simulink model "cdm"  (R2021a)
settings: Solver=VariableStepAuto  StartTime=0.0  StopTime=10  RelTol=1e-7
values from neighbouring files (symbols this model uses):
  A = [0 1; -8.31 -6.08]    [usv.m]
  B = [0; 8.31]    [usv.m]
  C = [1 0]    [usv.m]
  K = [0 0 1]*Con    [usv.m]
settings Model: Creator=lang  LastModifiedBy=lang

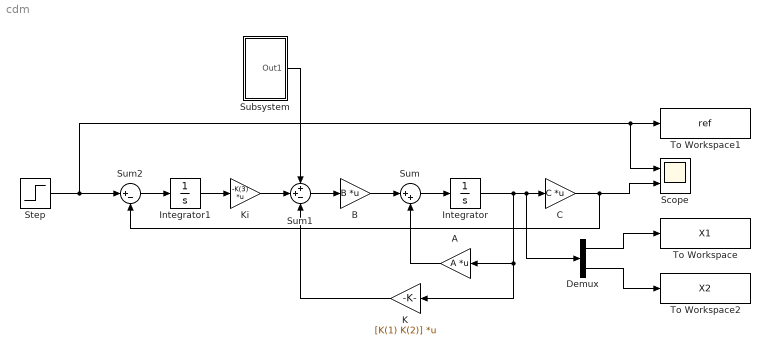
== system cdm ==
  A : Gain  Gain=A  Multiplication=Matrix(K*u)
  B : Gain  Gain=B  Multiplication=Matrix(K*u)
  C : Gain  Gain=C  Multiplication=Matrix(K*u)
  Demux : Demux  Outputs=2
  Integrator : Integrator
  Integrator1 : Integrator
  K : Gain  Gain=[K(1) K(2)]  Multiplication=Matrix(K*u)
  Ki : Gain  Gain=-K(3)  Multiplication=Matrix(K*u)
  Scope : Scope  NumInputPorts=2
  Step : Step  Time=0  After=angle  SampleTime=0
  Subsystem : Subsystem
  Sum : Sum  Inputs=|++
  Sum1 : Sum  Inputs=++-
  Sum2 : Sum  Inputs=|+-
  To Workspace : ToWorkspace  VariableName=X1  SampleTime=-1
  To Workspace1 : ToWorkspace  VariableName=ref  SampleTime=-1
  To Workspace2 : ToWorkspace  VariableName=X2  SampleTime=-1
  wires:
  B/1 -> Sum/1
  Sum/1 -> Integrator/1
  A/1 -> Sum/2
  Sum1/1 -> B/1
  Integrator/1 -> Demux/1, C/1, K/1, A/1
  C/1 -> Sum2/2, Scope/2
  Sum2/1 -> Integrator1/1
  Integrator1/1 -> Ki/1
  Step/1 -> Sum2/1, Scope/1, To Workspace1/1
  K/1 -> Sum1/3
  Ki/1 -> Sum1/2
  Subsystem/1(Out1) -> Sum1/1
  Demux/1 -> To Workspace/1
  Demux/2 -> To Workspace2/1

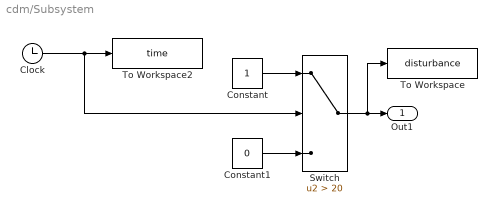
== system cdm/Subsystem ==
  Clock : Clock
  Constant : Constant
  Constant1 : Constant  Value=0
  Switch : Switch  Criteria=u2 > Threshold  Threshold=20
  To Workspace : ToWorkspace  VariableName=disturbance  SaveFormat=Timeseries  SampleTime=-1
  To Workspace2 : ToWorkspace  VariableName=time  SampleTime=-1
  Out1 : Outport
  wires:
  Constant1/1 -> Switch/3
  Constant/1 -> Switch/1
  Switch/1 -> To Workspace/1, Out1/1
  Clock/1 -> Switch/2, To Workspace2/1
